simulink model "modejer3a"  (Simulink 10.1)
settings: Solver=ode23s  StartTime=0.0  StopTime=60  RelTol=1e-3  EnableMultiTasking=on
values from neighbouring files (symbols this model uses):
  a = 0.05    [ejercicio2gain_scheduling.m]
  ciint = 0    [ejercicio2gain_scheduling.m]
  cix1 = 0    [ejercicio2gain_scheduling.m]
  cix2 = 0    [ejercicio2gain_scheduling.m]
  cix3 = 0    [ejercicio2gain_scheduling.m]
  g = 9.81    [ejercicio2gain_scheduling.m]
  k = 0.001    [ejercicio2gain_scheduling.m]
  L0 = 0.01    [ejercicio2gain_scheduling.m]
  L1 = 0.02    [ejercicio2gain_scheduling.m]
  m = 0.1    [ejercicio2gain_scheduling.m]
  pert = 0.04    [ejercicio2gain_scheduling.m]
  r = 1    [ejercicio2gain_scheduling.m]
libraries: simulink x1
settings Model: Creator=AP  LastModifiedBy=adpan
settings DataIOCC: LimitDataPoints=on  SignalLoggingSaveFormat=ModelDataLogs
settings OptimizationCC: ExpressionDepthLimit=2147483647  InitFltsAndDblsToZero=on
settings DebuggingCC: SaveWithParameterizedLinksMsg=none  SolverPrmCheckMsg=warning  FcnCallInpInsideContextMsg=warning  StateNameClashWarn=warning
settings SFSimCC: SimParseCustomCode=off
settings GRTTargetCC: TargetFcnLib=ansi_tfl_tmw.mat

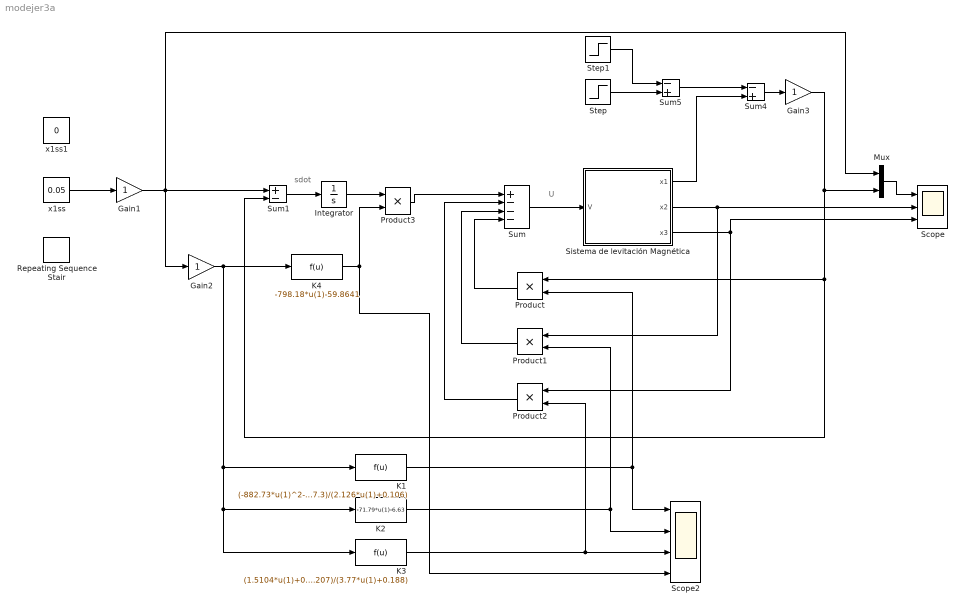
== system modejer3a ==
  note: U
  note: sdot
  Gain1 : Gain
  Gain2 : Gain
  Gain3 : Gain
  Integrator : Integrator  InitialCondition=ciint
  K1 : Fcn  Expr=(-882.73*u(1)^2-296.83*u(1)-17.3)/(2.126*u(1)+0.106)
  K2 : Fcn  Expr=-71.79*u(1)-6.63
  K3 : Fcn  Expr=(1.5104*u(1)+0.207)/(3.77*u(1)+0.188)
  K4 : Fcn  Expr=-798.18*u(1)-59.8641
  Mux : Mux  Inputs=2
  Product{,1..3} (4 alike) : Product  RndMeth=Zero
  Repeating Sequence Stair : simulink/Sources/Repeating Sequence Stair  OutValues=[0 0.02 0.04 0.06 0.08 0.1 0.12 0.14 0.16 0.18 0.2].'*3  tsamp=4  OutMin=[]  OutMax=[]  OutDataTypeStr=float('double')  OutputDataTypeScalingMode=Specify via dialog  OutDataType=float('double')  ConRadixGroup=Best Precision: Vector-wise  OutScaling=2^-12
  Scope : Scope  NumInputPorts=3
  Scope2 : Scope  NumInputPorts=4
  Sistema de levitación Magnética : Subsystem
  Step : Step  Time=5  After=pert  SampleTime=0
  Step1 : Step  Time=5.1  After=pert  SampleTime=0
  Sum : Sum  Inputs=+---
  Sum1 : Sum  Inputs=+-
  Sum4 : Sum  Inputs=-+
  Sum5 : Sum  Inputs=-+
  x1ss : Constant  Value=0.05
  x1ss1 : Constant  Value=0
  wires:
  Sistema de levitación Magnética/2(x2) -> Scope/2, Product1/1
  Sistema de levitación Magnética/3(x3) -> Product2/1, Scope/3
  Sum/1 -> Sistema de levitación Magnética/1(V)
  Product/1 -> Sum/4
  Product1/1 -> Sum/3
  Product2/1 -> Sum/2
  Gain3/1 -> Product/1, Sum1/2, Mux/2
  Sum4/1 -> Gain3/1
  Sistema de levitación Magnética/1(x1) -> Sum4/2
  Sum5/1 -> Sum4/1
  Step/1 -> Sum5/2
  Step1/1 -> Sum5/1
  Sum1/1 -> Integrator/1
  Product3/1 -> Sum/1
  Integrator/1 -> Product3/1
  K1/1 -> Product/2, Scope2/1
  K2/1 -> Product1/2, Scope2/2
  K3/1 -> Product2/2, Scope2/3
  K4/1 -> Product3/2, Scope2/4
  Gain1/1 -> Gain2/1, Sum1/1, Mux/1
  Gain2/1 -> K4/1, K1/1, K2/1, K3/1
  Mux/1 -> Scope/1
  x1ss/1 -> Gain1/1

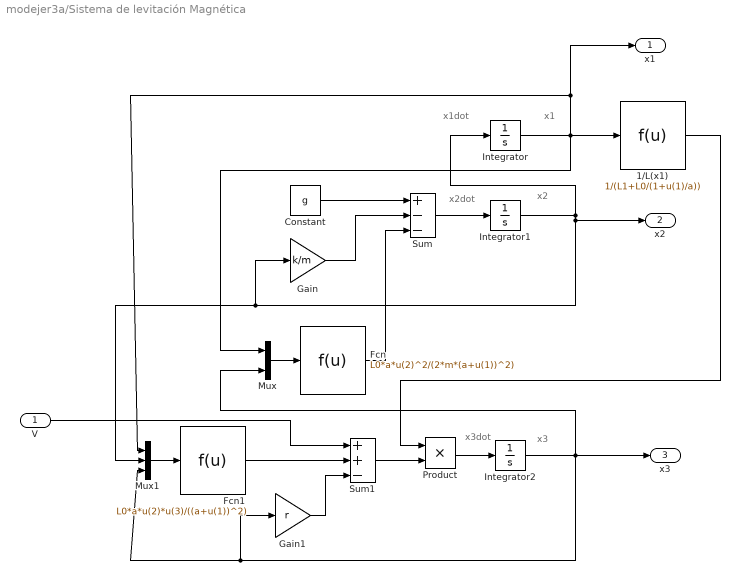
== system modejer3a/Sistema de levitación Magnética ==
  note: x1dot
  note: x1
  note: x2dot
  note: x2
  note: x3
  note: x3dot
  V : Inport
  1/L(x1) : Fcn  Expr=1/(L1+L0/(1+u(1)/a))
  Constant : Constant  Value=g
  Fcn : Fcn  Expr=L0*a*u(2)^2/(2*m*(a+u(1))^2)
  Fcn1 : Fcn  Expr=L0*a*u(2)*u(3)/((a+u(1))^2)
  Gain : Gain  Gain=k/m
  Gain1 : Gain  Gain=r
  Integrator : Integrator  InitialCondition=cix1
  Integrator1 : Integrator  InitialCondition=cix2
  Integrator2 : Integrator  InitialCondition=cix3
  Mux : Mux  Inputs=2
  Mux1 : Mux  Inputs=3
  Product : Product  RndMeth=Zero
  Sum : Sum  Inputs=+--
  Sum1 : Sum  Inputs=++-
  x1 : Outport
  x2 : Outport  Port=2
  x3 : Outport  Port=3
  wires:
  Sum/1 -> Integrator1/1
  Constant/1 -> Sum/1
  Gain/1 -> Sum/2
  Integrator1/1 -> Integrator/1, Gain/1, Mux1/2, x2/1
  Integrator/1 -> Mux/1, 1/L(x1)/1, Mux1/1, x1/1
  Mux/1 -> Fcn/1
  Integrator2/1 -> Mux/2, Gain1/1, Mux1/3, x3/1
  Fcn/1 -> Sum/3
  Product/1 -> Integrator2/1
  Sum1/1 -> Product/2
  1/L(x1)/1 -> Product/1
  Gain1/1 -> Sum1/3
  Mux1/1 -> Fcn1/1
  Fcn1/1 -> Sum1/2
  V/1 -> Sum1/1
